simulink model "matlab_to_backend_connection"  (R2024b)
settings: Solver=FixedStepDiscrete  StartTime=0.0  StopTime=inf  RelTol=1e-3  EnableMultiTasking=on
libraries: raspberrypiNetworklib x2
settings Model: ModifiedByFormat=The MathWorks Inc.  ExtModeTrigDuration=2  Creator=The MathWorks, Inc.  LastModifiedBy=The MathWorks Inc.
settings SolverCC: AlgebraicLoopSolver=TrustRegion  PositivePriorityOrder=on  MaxZcPerStep=1
settings DataIOCC: LimitDataPoints=on  SaveFormat=Array  ReturnWorkspaceOutputs=off
settings OptimizationCC: LifeSpan=1  MaxStackSize=200000  EfficientTunableParamExpr=on
settings DebuggingCC: UnderspecifiedInitializationDetection=Classic  MergeDetectMultiDrivingBlocksExec=none  SolverPrmCheckMsg=warning  UnconnectedInputMsg=warning  UnconnectedOutputMsg=warning  UnconnectedLineMsg=warning  AllowSymbolicDim=off  SFUnexpectedBacktrackingDiag=warning  SFNoUnconditionalDefaultTransitionDiag=warning  SFExecutionAtInitializationDiag=none  ArithmeticOperatorsInVariantConditions=warning
settings HardwareCC: ProdBitPerPointer=32  ProdBitPerSizeT=32  ProdBitPerPtrDiffT=32  ProdLargestAtomicInteger=Long  ProdLargestAtomicFloat=Double  ProdWordSize=32  ProdLongLongMode=on  ProdHWDeviceType=ARM Compatible->ARM Cortex-A (32-bit)
settings ModelReferenceCC: EnableRefExpFcnMdlSchedulingChecks=on  PropagateSignalLabelsOutOfModel=off
settings SFSimCC: SimUseLocalCustomCode=off  CustomCodeUndefinedFunction=UseInterfaceOnly
settings RTWCC: Description=Embedded Coder  SystemTargetFile=ert.tlc  HardwareBoard=Raspberry Pi  TLCOptions="-aInlineSetEventsForThisBaseRateFcn=TLC_FALSE -aSuppressMultiTaskScheduler=TLC_FALSE  -aRateBasedStepFcn=0"  TemplateMakefile=ert_default_tmf  RTWUseLocalCustomCode=off  Toolchain=GNU GCC Embedded Linux  BuildConfiguration=Faster Runs  GPUComputeCapability=3.5  DLArmComputeVersion=19.05
settings CodeAppCC: IgnoreCustomStorageClasses=off  StateflowObjectComments=on
settings ERTTargetCC: CodeReplacementLibrary=ARM Cortex-A CMSIS  MultiwordLength=2048  SupportVariableSizeSignals=on  ExtModeTransport=2  ExtModeStaticAlloc=on  ExtModeMexFile=ext_xcp  ExtModeIntrfLevel=Level2 - Open  InlinedParameterPlacement=Hierarchical  ConvertIfToSwitch=off  SuppressUnreachableDefaultCases=off  DynamicArrayContainerType=coder::array
settings ConfigComp: CovMetricSettings=dw  CovSaveCumulativeToWorkspaceVar=on  CovSaveSingleToWorkspaceVar=on  CovExternalEMLEnable=off  CovSFcnEnable=off

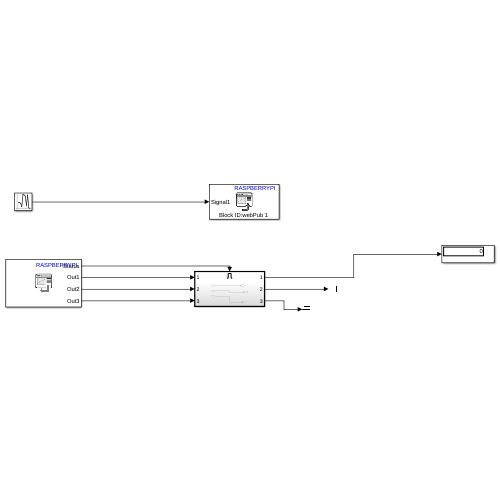
[thumbnail: Simulink's stored preview of the top-level diagram]
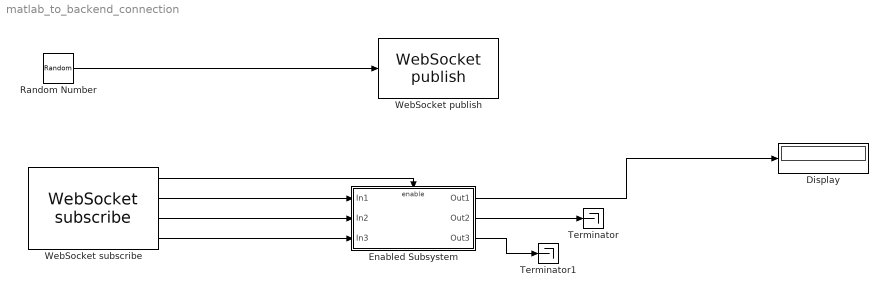
== system matlab_to_backend_connection ==
  Display : Display
  Enabled Subsystem : Subsystem  TreatAsAtomicUnit=on
  Random Number : RandomNumber  SampleTime=0.1
  Terminator : Terminator
  Terminator1 : Terminator
  WebSocket publish : raspberrypiNetworklib/WebSocket publish  UniqueBlockID=webPub 1  IPAddress=172.16.16.70  Port=8080  NumberOfSignals=1  webSocketId=matlab_to_backend_connection/WebSocket_publish  BlockPlatform=RASPBERRYPI
  WebSocket subscribe : raspberrypiNetworklib/WebSocket subscribe  IPAddress=172.16.16.70  Port=8080  OutputCfg=Mask Dialog  numSignals=3  Dsize1=1  Dtype1=single  Dsize2=1  Dtype2=single  Dsize3=1  Dtype3=single  Dsize4=1  Dtype4=double  Dsize5=1  Dtype5=double  Dsize6=1  Dtype6=double  Dsize7=1  Dtype7=double  Dsize8=1  Dtype8=double  Dsize9=1  Dtype9=double  Dsize10=1  Dtype10=double  Sampletime=0.1  NumberOfSignals=3  webSocketId=matlab_to_backend_connection/WebSocket_subscribe  BlockPlatform=RASPBERRYPI
  wires:
  Random Number/1 -> WebSocket publish/1
  WebSocket subscribe/1 -> Enabled Subsystem/Enable
  WebSocket subscribe/2 -> Enabled Subsystem/1(In1)
  Enabled Subsystem/1(Out1) -> Display/1
  WebSocket subscribe/3 -> Enabled Subsystem/2(In2)
  WebSocket subscribe/4 -> Enabled Subsystem/3(In3)
  Enabled Subsystem/2(Out2) -> Terminator/1
  Enabled Subsystem/3(Out3) -> Terminator1/1

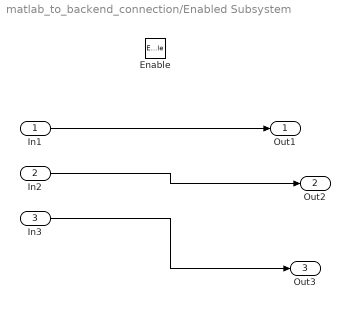
== system matlab_to_backend_connection/Enabled Subsystem ==
  In1 : Inport
  In2 : Inport  Port=2
  In3 : Inport  Port=3
  Enable : EnablePort
  Out1 : Outport
  Out2 : Outport  Port=2
  Out3 : Outport  Port=3
  wires:
  In1/1 -> Out1/1
  In2/1 -> Out2/1
  In3/1 -> Out3/1
